simulink model "FotoTParam"  (R2021a)
settings: Solver=VariableStepAuto  StartTime=-10  StopTime=10  RelTol=1e-3
libraries: aerolibconvert2 x4
settings Model: OrderedModelArguments=off  Creator=Siro  LastModifiedBy=Siro

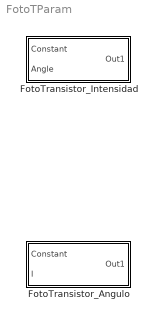
== system FotoTParam ==
  FotoTransistor_Angulo : Subsystem
  FotoTransistor_Intensidad : Subsystem

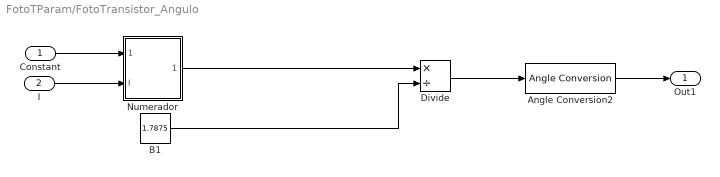
== system FotoTParam/FotoTransistor_Angulo ==
  Constant : Inport
  I : Inport  Port=2
  Angle Conversion2 : aerolibconvert2/Angle Conversion  IU=rad  OU=deg
  B1 : Constant  Value=1.7875
  Divide : Product  Inputs=*/
  Numerador : Subsystem
  Out1 : Outport
  wires:
  B1/1 -> Divide/2
  Constant/1 -> Numerador/1(Constant)
  I/1 -> Numerador/2(I)
  Numerador/1(Out1) -> Divide/1
  Divide/1 -> Angle Conversion2/1
  Angle Conversion2/1 -> Out1/1

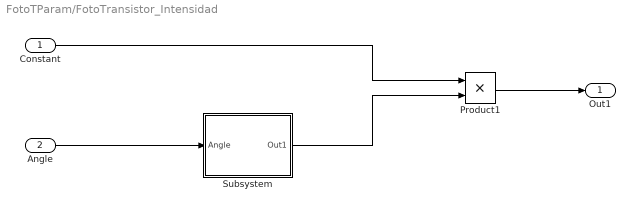
== system FotoTParam/FotoTransistor_Intensidad ==
  Constant : Inport
  Angle : Inport  Port=2
  Product1 : Product
  Subsystem : Subsystem
  Out1 : Outport
  wires:
  Angle/1 -> Subsystem/1(Angle)
  Constant/1 -> Product1/1
  Subsystem/1(Out1) -> Product1/2
  Product1/1 -> Out1/1

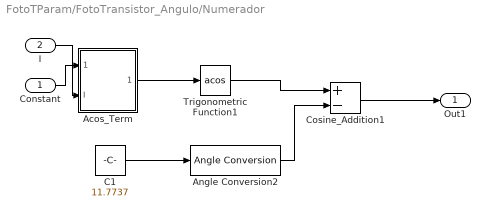
== system FotoTParam/FotoTransistor_Angulo/Numerador ==
  Constant : Inport
  I : Inport  Port=2
  Acos_Term : Subsystem
  Angle Conversion2 : aerolibconvert2/Angle Conversion  IU=deg  OU=rad
  C1 : Constant  Value=11.7737
  Cosine_Addition1 : Sum  Inputs=+-
  Trigonometric Function1 : Trigonometry  Operator=acos
  Out1 : Outport
  wires:
  Angle Conversion2/1 -> Cosine_Addition1/2
  Trigonometric Function1/1 -> Cosine_Addition1/1
  C1/1 -> Angle Conversion2/1
  Constant/1 -> Acos_Term/1(Constant)
  Acos_Term/1(Out1) -> Trigonometric Function1/1
  I/1 -> Acos_Term/2(I)
  Cosine_Addition1/1 -> Out1/1

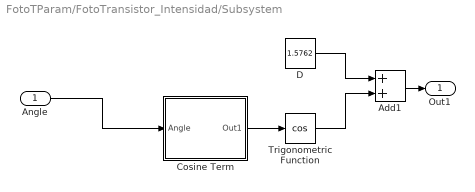
== system FotoTParam/FotoTransistor_Intensidad/Subsystem ==
  Angle : Inport
  Add1 : Sum
  Cosine Term : Subsystem
  D : Constant  Value=1.5762
  Trigonometric Function : Trigonometry  Operator=cos
  Out1 : Outport
  wires:
  Cosine Term/1(Out1) -> Trigonometric Function/1
  Angle/1 -> Cosine Term/1(Angle)
  Add1/1 -> Out1/1
  Trigonometric Function/1 -> Add1/2
  D/1 -> Add1/1

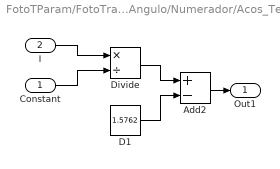
== system FotoTParam/FotoTransistor_Angulo/Numerador/Acos_Term ==
  Constant : Inport
  I : Inport  Port=2
  Add2 : Sum  Inputs=+-
  D1 : Constant  Value=1.5762
  Divide : Product  Inputs=*/
  Out1 : Outport
  wires:
  Divide/1 -> Add2/1
  D1/1 -> Add2/2
  Constant/1 -> Divide/2
  I/1 -> Divide/1
  Add2/1 -> Out1/1

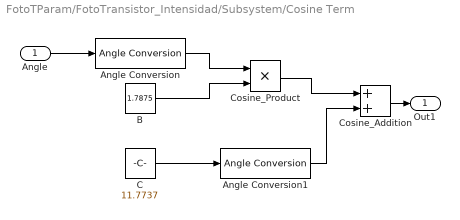
== system FotoTParam/FotoTransistor_Intensidad/Subsystem/Cosine Term ==
  Angle : Inport
  Angle Conversion : aerolibconvert2/Angle Conversion  IU=deg  OU=rad
  Angle Conversion1 : aerolibconvert2/Angle Conversion  IU=deg  OU=rad
  B : Constant  Value=1.7875
  C : Constant  Value=11.7737
  Cosine_Addition : Sum
  Cosine_Product : Product
  Out1 : Outport
  wires:
  Angle/1 -> Angle Conversion/1
  B/1 -> Cosine_Product/2
  Angle Conversion/1 -> Cosine_Product/1
  Cosine_Product/1 -> Cosine_Addition/1
  Cosine_Addition/1 -> Out1/1
  C/1 -> Angle Conversion1/1
  Angle Conversion1/1 -> Cosine_Addition/2
